simulink model "BuckConverterLinearModel"  (R2020a)
settings: Solver=ode23s  StartTime=0.0  StopTime=0.6  RelTol=1e-3
values from neighbouring files (symbols this model uses):
  C = 3000e-6    (= 0.003)    [parameter.m]
  L = 500*10^-6    (= 0.0005)    [parameter.m]
  Load = 1    [parameter.m]
  RL = 10e-3    (= 0.01)    [parameter.m]
settings Model: Creator=ykamatan  LastModifiedBy=ykamatan

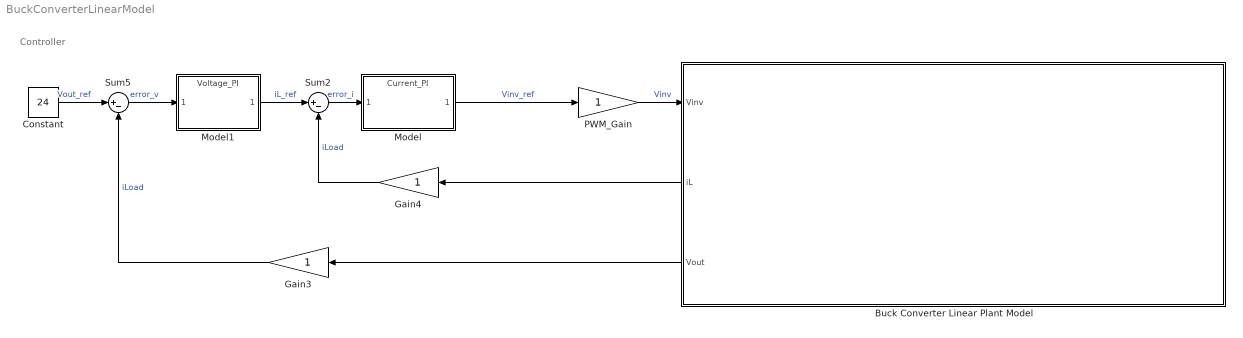
== system BuckConverterLinearModel ==
  note: Controller
  Buck Converter Linear Plant Model : Subsystem
      settings: PortSchema="{\"entries\":[{\"content\":{\"sides\":[{\"content\":{\"connectorIds\":[\"In1\",\"Out1\",\"Out2\"]},\"type\":\"ConnectorPlacement.EquallySpacedRectSide\",\"uuid\":\"b66999c5-eb46-47e5-8c3d-17284b7a3d16\"},{\"content\":{\"connectorIds\":[],\"side\":\"RIGHT\"},\"type\":\"ConnectorPlacement.EquallySpacedRectSide\",\"uuid\":\"17d4eac5-cf5c-4a79-9618-dbb8569cb044\"},{\"content\":{\"connectorIds\":[],\"side\":\"TOP\"},\"type\":\"ConnectorPlacement.EquallySpacedRectSide\",\"uuid\":\"07f337b7-51df-4226-bcf0-2b6cd1bf51b5\"}]},\"type\":\"ConnectorPlacement.EquallySpacedConnector\",\"uuid\":\"76f1c238-310f-49e4-b895-c8ccad5ae75f\"}],\"packageUris\":[\"http://schema.mathworks.com/mf0/Connector/19700101\"],\"version\":\"1.0\"}"
  Constant : Constant  Value=24
  Gain3 : Gain
  Gain4 : Gain
  Model : ModelReference  ModelNameDialog=Current_PI.slx  SimulationMode=Normal  ModelReferenceVersion=1.10
  Model1 : ModelReference  ModelNameDialog=Voltage_PI.slx  SimulationMode=Normal  ModelReferenceVersion=1.10
  PWM_Gain : Gain
  Sum2 : Sum  Inputs=|+-
  Sum5 : Sum  Inputs=|+-
  wires:
  Constant/1 -> Sum5/1  "Vout_ref"
  Sum2/1 -> Model/1  "error_i"
  Model/1 -> PWM_Gain/1  "Vinv_ref"
  Sum5/1 -> Model1/1  "error_v"
  Gain4/1 -> Sum2/2  "iLoad"
  Gain3/1 -> Sum5/2  "iLoad"
  Model1/1 -> Sum2/1  "iL_ref"
  PWM_Gain/1 -> Buck Converter Linear Plant Model/1(Vinv)  "Vinv"
  Buck Converter Linear Plant Model/1(iL) -> Gain4/1
  Buck Converter Linear Plant Model/2(Vout) -> Gain3/1

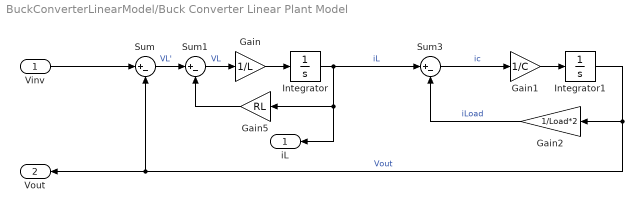
== system BuckConverterLinearModel/Buck Converter Linear Plant Model ==
  Vinv : Inport
  Gain : Gain  Gain=1/L
  Gain1 : Gain  Gain=1/C
  Gain2 : Gain  Gain=1/Load*2
  Gain5 : Gain  Gain=RL
  Integrator : Integrator
  Integrator1 : Integrator
  Sum : Sum  Inputs=|+-
  Sum1 : Sum  Inputs=|+-
  Sum3 : Sum  Inputs=|+-
  iL : Outport
  Vout : Outport  Port=2
  wires:
  Gain/1 -> Integrator/1
  Gain1/1 -> Integrator1/1
  Gain5/1 -> Sum1/2
  Integrator1/1 -> Vout/1, Sum/2, Gain2/1  "Vout"
  Sum/1 -> Sum1/1  "VL'"
  Gain2/1 -> Sum3/2  "iLoad"
  Sum3/1 -> Gain1/1  "ic"
  Integrator/1 -> Sum3/1, iL/1, Gain5/1  "iL"
  Sum1/1 -> Gain/1  "VL"
  Vinv/1 -> Sum/1
